simulink model "BatteryElectricWholeModel"  (R2024a)
settings: Solver=VariableStepAuto  StartTime=0.0  StopTime=10.0  RelTol=1e-3
settings Model: Creator=44779  LastModifiedBy=44779

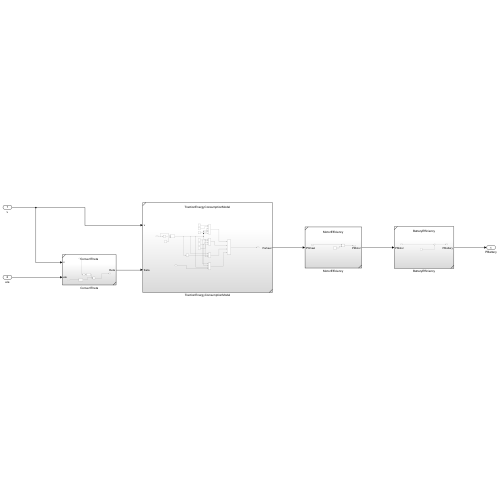
[thumbnail: Simulink's stored preview of the top-level diagram]
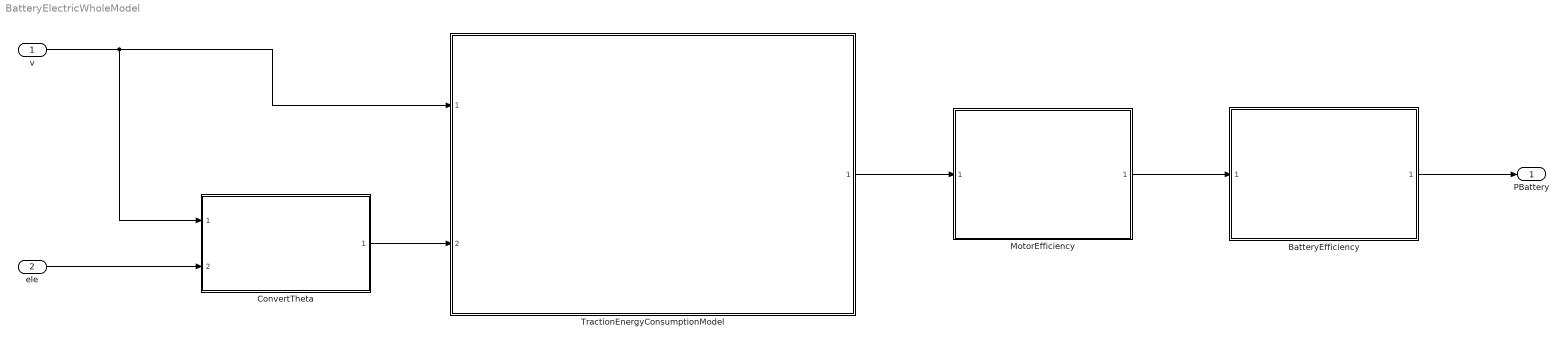
== system BatteryElectricWholeModel ==
  v : Inport
  ele : Inport  Port=2
  BatteryEfficiency : Subsystem  ReferencedSubsystem=BatteryEfficiency
  ConvertTheta : Subsystem  ReferencedSubsystem=ConvertTheta
  MotorEfficiency : Subsystem  ReferencedSubsystem=MotorEfficiency
  TractionEnergyConsumptionModel : Subsystem  ReferencedSubsystem=TractionEnergyConsumptionModel
  PBattery : Outport
  wires:
  v/1 -> ConvertTheta/1, TractionEnergyConsumptionModel/1
  TractionEnergyConsumptionModel/1 -> MotorEfficiency/1
  MotorEfficiency/1 -> BatteryEfficiency/1
  BatteryEfficiency/1 -> PBattery/1
  ele/1 -> ConvertTheta/2
  ConvertTheta/1 -> TractionEnergyConsumptionModel/2
